simulink model "adcs_controller"  (R2024b)
settings: Solver=VariableStepAuto  StartTime=0.0  StopTime=10.0  RelTol=1e-3
undefined symbols (not defined in the file): K_lqr
settings Model: DataDictionary=adcs_params.sldd  Creator=natha  LastModifiedBy=natha

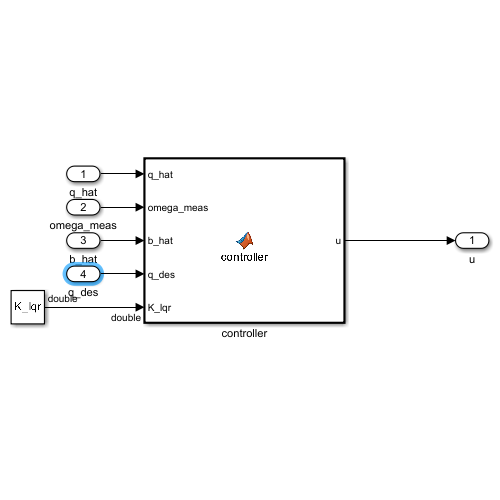
[thumbnail: Simulink's stored preview of the top-level diagram]
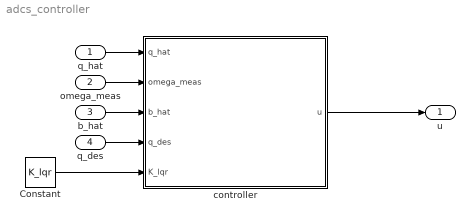
== system adcs_controller ==
  q_hat : Inport  PortDimensions=4
  omega_meas : Inport  Port=2  PortDimensions=3
  b_hat : Inport  Port=3  PortDimensions=3
  q_des : Inport  Port=4  PortDimensions=4
  Constant : Constant  Value=K_lqr
  controller : MATLAB Function  TreatAsAtomicUnit=on
  u : Outport  PortDimensions=[3 1]
  wires:
  controller/1(u) -> u/1
  q_hat/1 -> controller/1(q_hat)
  omega_meas/1 -> controller/2(omega_meas)
  b_hat/1 -> controller/3(b_hat)
  q_des/1 -> controller/4(q_des)
  Constant/1 -> controller/5(K_lqr)

== matlab function adcs_controller/controller ==
  data: q_hat input; u output; omega_meas input; b_hat input; q_des input; K_lqr input
function u = controller(q_hat, omega_meas, b_hat, q_des, K_lqr)
    q_des_conj = [-q_des(1); -q_des(2); -q_des(3); q_des(4)];
    dq = quatmultiply(q_hat, q_des_conj);
    delta_theta = 2*dq(1:3);
    omega_hat = omega_meas - b_hat;
    x = [delta_theta; omega_hat];
    u = -K_lqr*x;
end

function pq = quatmultiply(p,q)
    pq = [ p(4)*q(1) + p(3)*q(2) - p(2)*q(3) + p(1)*q(4);
          -p(3)*q(1) + p(4)*q(2) + p(1)*q(3) + p(2)*q(4);
           p(2)*q(1) - p(1)*q(2) + p(4)*q(3) + p(3)*q(4);
          -p(1)*q(1) - p(2)*q(2) - p(3)*q(3) + p(4)*q(4) ];
end
